simulink model "COM_BancMonitor"  (Simulink 8.6)
settings: Solver=FixedStepDiscrete  StartTime=0.0  StopTime=inf  FixedStep=ComMinSampleTime  RelTol=1e-3
values from neighbouring files (symbols this model uses):
  ComMinSampleTime = 1/400    (= 0.0025)    [init_BancMonitor.m]
  g = 9.81    [init_BancMonitor.m]
  LandingHeight = 0.08    [init_BancMonitor.m]
  Ts_AttitudeLoop = 1/200    (= 0.005)    [init_BancMonitor.m]
  Ts_PositionLoop = 1/100    (= 0.01)    [init_BancMonitor.m]
undefined symbols (not defined in the file or in its folder): a_PWM, b_PWM, BiasAcc, DiscIntNeverNeededParam, Gumstix, m, MaxThrottle, MinThrottle, MPU6050, PositionSecuMax, PositionSecuMin, Tacc, time_unfolding, Tmax, Tmin, TorquesSat, UAVstruct
undefined symbols (not defined in the file): AccMax, AccMaxScenario, AccMin, AccMinScenario, b_est0, dc_open, PositionMax, PositionMin, SpeedMax, SpeedMaxScenario, SpeedMin, SpeedMinScenario, Ts_detector, Ts_Wifi
libraries: simulink x34, custom_lib x27, simulink_extras x11
(part 2 of 3)

== system COM_BancMonitor/GUMSTIX/DETECTOR_PARAMETERS ==
  Max_no_detection : Constant  Value=5  OutDataTypeStr=Inherit: Inherit via back propagation  SampleTime=-1
  Mux6 : Mux  Inputs=[2 2 2 4 2 4 2 4]
  bin_square : Constant  Value=100  OutDataTypeStr=Inherit: Inherit via back propagation  SampleTime=-1
  blur_size : Constant  Value=3  OutDataTypeStr=Inherit: Inherit via back propagation  SampleTime=-1
  float32 to uint8 (BE) : custom_lib/CONVERTERS/float32 to uint8 (BE)
  float32 to uint8 (BE)1 : custom_lib/CONVERTERS/float32 to uint8 (BE)
  float32 to uint8 (BE)2 : custom_lib/CONVERTERS/float32 to uint8 (BE)
  k_approx : Constant  Value=0.02  OutDataTypeStr=Inherit: Inherit via back propagation  SampleTime=-1
  thresh_area : Constant  Value=1000  OutDataTypeStr=Inherit: Inherit via back propagation  SampleTime=-1
  thresh_cos : Constant  Value=0.1  OutDataTypeStr=Inherit: Inherit via back propagation  SampleTime=-1
  thresh_diff : Constant  Value=20*20  OutDataTypeStr=Inherit: Inherit via back propagation  SampleTime=-1
  thresh_ratio : Constant  Value=0.2  OutDataTypeStr=Inherit: Inherit via back propagation  SampleTime=-1
  uint16 to uint8 (BE){,1..4} (5 alike) : custom_lib/CONVERTERS/uint16 to uint8 (BE)
  Detector_param : Outport
  wires:
  Mux6/1 -> Detector_param/1
  thresh_ratio/1 -> float32 to uint8 (BE)2/1
  k_approx/1 -> float32 to uint8 (BE)/1
  thresh_area/1 -> uint16 to uint8 (BE)2/1
  thresh_cos/1 -> float32 to uint8 (BE)1/1
  thresh_diff/1 -> uint16 to uint8 (BE)3/1
  float32 to uint8 (BE)/1 -> Mux6/4
  float32 to uint8 (BE)1/1 -> Mux6/6
  float32 to uint8 (BE)2/1 -> Mux6/8
  blur_size/1 -> uint16 to uint8 (BE)1/1
  bin_square/1 -> uint16 to uint8 (BE)/1
  uint16 to uint8 (BE)2/1 -> Mux6/5
  uint16 to uint8 (BE)3/1 -> Mux6/7
  uint16 to uint8 (BE)1/1 -> Mux6/2
  uint16 to uint8 (BE)/1 -> Mux6/3
  Max_no_detection/1 -> uint16 to uint8 (BE)4/1
  uint16 to uint8 (BE)4/1 -> Mux6/1

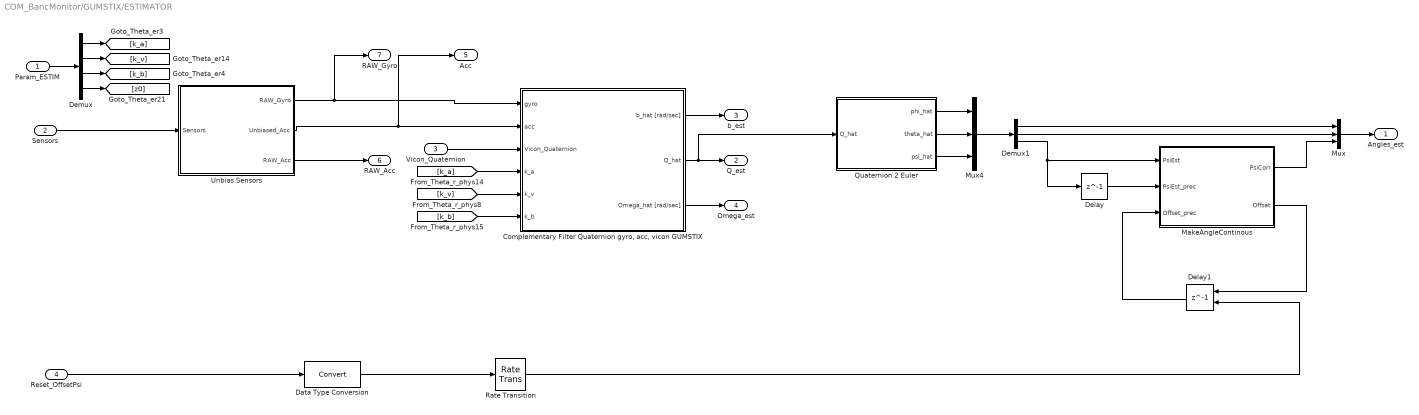
== system COM_BancMonitor/GUMSTIX/ESTIMATOR ==
  Param_ESTIM : Inport
  Sensors : Inport  Port=2
  Vicon_Quaternion : Inport  Port=3
  Reset_OffsetPsi : Inport  Port=4
  "Complementary Filter Quaternion gyro, acc, vicon GUMSTIX" : Subsystem  mask(COMPLEMENTARY FILTER){Ts_param=Ts_AttitudeLoop, b0_param=single(b_est0), Q0_param=single([1;0;0;0]), acc_ref_param=single([0;0;-g])}
      mask prompts: Ts_param "Sample Time [s]"; b0_param "Initial bias [deg/s]"; Q0_param "Initial Quaternion"; acc_ref_param "Accelerometer Reference"
      mask help:
      | This block assure a complementary filtering of IMU's data and vicon's data.
      |
      | ka: the gain to adjust accelerometer's sensibility
      |     A digonal matrix [3x3]:
      | kv: the gain to adjust vicon's sensibility
      |     A digonal matrix [3x3]
      | kb: the gain to adjust the bias sensibility
      |     A digonal matrix [3x3]
      |
      | Remark: For each diagonal matrix gain:
      |     - kx(1,1) = roll sensibilty
      |     - kx(2,2) = pitch sensibilty
      |     - kx(3,3) = yaw sensibilty
  Data Type Conversion : DataTypeConversion
  Delay : Delay  DelayLength=1
  Delay1 : Delay  DelayLength=1  ExternalReset=Level hold
      settings: InputPortMap=u0,r5
  Demux : Demux  Outputs=[3; 3; 3; 1]
  Demux1 : Demux  Outputs=3
  MakeAngleContinous : MATLAB Function  TreatAsAtomicUnit=on
  Mux : Mux  Inputs=3
  Mux4 : Mux  Inputs=3
  Quaternion 2 Euler : MATLAB Function  TreatAsAtomicUnit=on
  Rate Transition : RateTransition
  Unbias Sensors : Subsystem
  Angles_est : Outport
  Q_est : Outport  Port=2
  b_est : Outport  Port=3
  Omega_est : Outport  Port=4
  Acc : Outport  Port=5
  RAW_Acc : Outport  Port=6
  RAW_Gyro : Outport  Port=7
  wires:
  Sensors/1 -> Unbias Sensors/1(Sensors)
  Unbias Sensors/2(Unbiased_Acc) -> Acc/1, "Complementary Filter Quaternion gyro, acc, vicon GUMSTIX"/2(acc)
  Unbias Sensors/1(RAW_Gyro) -> "Complementary Filter Quaternion gyro, acc, vicon GUMSTIX"/1(gyro), RAW_Gyro/1
  "Complementary Filter Quaternion gyro, acc, vicon GUMSTIX"/1(b_hat [rad/sec]) -> b_est/1
  [k_a] -> "Complementary Filter Quaternion gyro, acc, vicon GUMSTIX"/4(k_a)
  "Complementary Filter Quaternion gyro, acc, vicon GUMSTIX"/2(Q_hat) -> Q_est/1, Quaternion 2 Euler/1(Q_hat)
  [k_v] -> "Complementary Filter Quaternion gyro, acc, vicon GUMSTIX"/5(k_v)
  [k_b] -> "Complementary Filter Quaternion gyro, acc, vicon GUMSTIX"/6(k_b)
  Param_ESTIM/1 -> Demux/1
  Demux/1 -> [k_a]
  Demux/2 -> [k_v]
  Demux/3 -> [k_b]
  Demux/4 -> [z0]
  Vicon_Quaternion/1 -> "Complementary Filter Quaternion gyro, acc, vicon GUMSTIX"/3(Vicon_Quaternion)
  Delay/1 -> MakeAngleContinous/2(PsiEst_prec)
  Delay1/1 -> MakeAngleContinous/3(Offset_prec)
  MakeAngleContinous/2(Offset) -> Delay1/1
  Mux/1 -> Angles_est/1
  Demux1/3 -> Delay/1, MakeAngleContinous/1(PsiEst)
  Demux1/2 -> Mux/2
  Demux1/1 -> Mux/1
  MakeAngleContinous/1(PsiCorr) -> Mux/3
  Reset_OffsetPsi/1 -> Data Type Conversion/1
  Rate Transition/1 -> Delay1/2
  Data Type Conversion/1 -> Rate Transition/1
  Unbias Sensors/3(RAW_Acc) -> RAW_Acc/1
  Quaternion 2 Euler/1(phi_hat) -> Mux4/1
  Quaternion 2 Euler/2(theta_hat) -> Mux4/2
  Quaternion 2 Euler/3(psi_hat) -> Mux4/3
  Mux4/1 -> Demux1/1
  "Complementary Filter Quaternion gyro, acc, vicon GUMSTIX"/3(Omega_hat [rad/sec]) -> Omega_est/1

== system COM_BancMonitor/GUMSTIX/ESTIMATOR_PARAMETERS ==
  Mux1 : Mux  Inputs=2
  Mux6 : Mux  Inputs=3
  Time Constant Gyro Filter : Constant  Value=0.3897 %exp(-2*pi*30*ComMinSampleTime)  OutDataTypeStr=Inherit: Inherit via back propagation  SampleTime=-1
  k_a : Constant  Value=[.4 .4 0]  OutDataTypeStr=Inherit: Inherit via back propagation  SampleTime=-1
  k_b : Constant  Value=[.08 .08 .08]  OutDataTypeStr=Inherit: Inherit via back propagation  SampleTime=-1
  k_v : Constant  Value=[0 0 2]  OutDataTypeStr=Inherit: Inherit via back propagation  SampleTime=-1
  Est_Param : Outport
  wires:
  k_a/1 -> Mux6/1
  k_b/1 -> Mux6/3
  k_v/1 -> Mux6/2
  Mux6/1 -> Mux1/1
  Time Constant Gyro Filter/1 -> Mux1/2
  Mux1/1 -> Est_Param/1

== system COM_BancMonitor/GUMSTIX/Manual_Controller ==
  RX_Data : Inport
  Angles_est : Inport  Port=2
  Gyo Acc2 : Mux  Inputs=[1 1 1]
  In_from_UDP_Demux1 : Demux  Outputs=3
  In_from_UDP_Demux3 : Demux  Outputs=[1 1 1 1]
  Product : Product  Inputs=*/  RndMeth=Zero
  Product1 : Product  Inputs=**  RndMeth=Zero
  RX Angles Ref  Generator : Subsystem
  Saturation1 : Saturate  UpperLimit=Tmax*9.81*4  LowerLimit=Tmin*9.81*4
  Terminator : Terminator
  Trigonometric Function : Trigonometry  Operator=cos
  Trigonometric Function1 : Trigonometry  Operator=cos
  Angles_ref : Outport
  Thrust_ref : Outport  Port=2
  wires:
  RX Angles Ref  Generator/1(Roll_ref) -> Gyo Acc2/1
  RX Angles Ref  Generator/2(Pitch_ref) -> Gyo Acc2/2
  RX Angles Ref  Generator/3(Yaw_ref) -> Gyo Acc2/3
  Angles_est/1 -> In_from_UDP_Demux1/1
  Product1/1 -> Product/2
  In_from_UDP_Demux1/1 -> Trigonometric Function/1
  In_from_UDP_Demux1/2 -> Trigonometric Function1/1
  In_from_UDP_Demux1/3 -> Terminator/1
  Trigonometric Function1/1 -> Product1/2
  Trigonometric Function/1 -> Product1/1
  RX Angles Ref  Generator/4(Throttle_ref) -> Product/1
  Product/1 -> Saturation1/1
  Saturation1/1 -> Thrust_ref/1
  In_from_UDP_Demux3/1 -> RX Angles Ref  Generator/1(Roll_RX)
  In_from_UDP_Demux3/2 -> RX Angles Ref  Generator/2(Pitch_RX)
  In_from_UDP_Demux3/3 -> RX Angles Ref  Generator/3(Yaw_RX)
  In_from_UDP_Demux3/4 -> RX Angles Ref  Generator/4(Throttle_RX)
  RX_Data/1 -> In_from_UDP_Demux3/1
  Gyo Acc2/1 -> Angles_ref/1

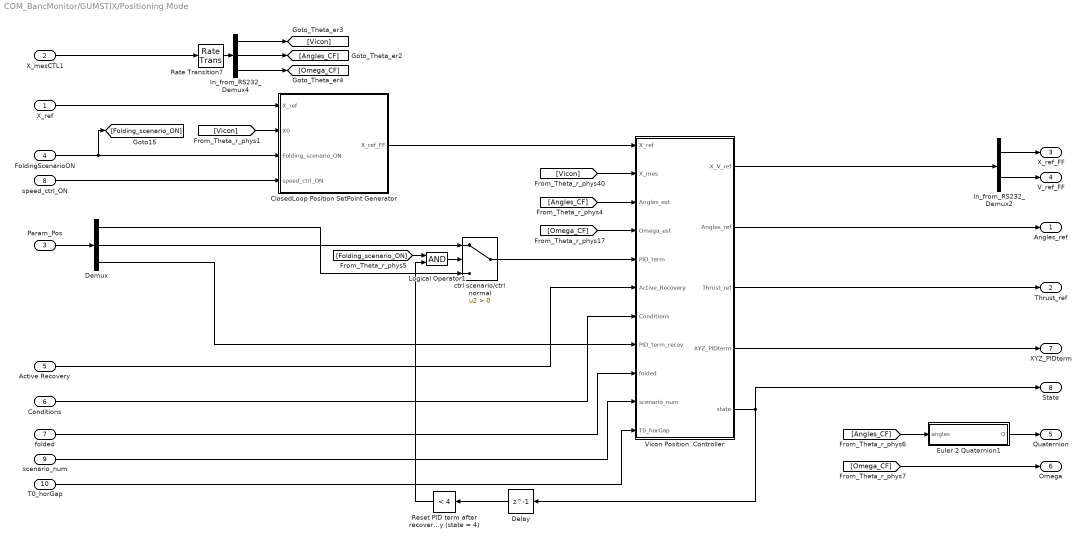
== system COM_BancMonitor/GUMSTIX/Positioning Mode ==
  X_ref : Inport
  X_mesCTL1 : Inport  Port=2
  Param_Pos : Inport  Port=3
  FoldingScenarioON : Inport  Port=4
  Active Recovery : Inport  Port=5
  Conditions : Inport  Port=6
  folded : Inport  Port=7
  speed_ctrl_ON : Inport  Port=8
  scenario_num : Inport  Port=9
  T0_horGap : Inport  Port=10
  ClosedLoop Position SetPoint Generator : Subsystem
  Delay : Delay  DelayLength=1  InitialCondition=0
  Demux : Demux  Outputs=[12 12 12]
  Euler 2 Quaternion1 : MATLAB Function  TreatAsAtomicUnit=on
  In_from_RS232_Demux2 : Demux  Outputs=[3 3]
  In_from_RS232_Demux4 : Demux  Outputs=[6 3 3]
  Logical Operator1 : Logic  AllPortsSameDT=off  OutDataTypeStr=boolean
  Rate Transition7 : RateTransition  OutPortSampleTime=Ts_PositionLoop
  Reset PID term after recovery (state = 4) : simulink/Logic and Bit Operations/Compare To Constant  relop=<  const=4  OutDataTypeStr=boolean
  Vicon Position  Controller : Subsystem
  ctrl scenario/ctrl normal : Switch  Criteria=u2 > Threshold
  Angles_ref : Outport
  Thrust_ref : Outport  Port=2
  X_ref_FF : Outport  Port=3
  V_ref_FF : Outport  Port=4
  Quaternion : Outport  Port=5
  Omega : Outport  Port=6
  XYZ_PIDterm : Outport  Port=7
  State : Outport  Port=8
  wires:
  [Vicon] -> Vicon Position  Controller/2(X_mes)
  [Vicon] -> ClosedLoop Position SetPoint Generator/2(X0)
  ClosedLoop Position SetPoint Generator/1(X_ref_FF) -> Vicon Position  Controller/1(X_ref)
  In_from_RS232_Demux2/1 -> X_ref_FF/1
  In_from_RS232_Demux2/2 -> V_ref_FF/1
  Vicon Position  Controller/1(X_V_ref) -> In_from_RS232_Demux2/1
  In_from_RS232_Demux4/1 -> [Vicon]
  In_from_RS232_Demux4/2 -> [Angles_CF]
  [Angles_CF] -> Vicon Position  Controller/3(Angles_est)
  Euler 2 Quaternion1/1(Q) -> Quaternion/1
  [Omega_CF] -> Omega/1
  In_from_RS232_Demux4/3 -> [Omega_CF]
  X_mesCTL1/1 -> Rate Transition7/1
  Rate Transition7/1 -> In_from_RS232_Demux4/1
  Vicon Position  Controller/4(XYZ_PIDterm) -> XYZ_PIDterm/1
  FoldingScenarioON/1 -> ClosedLoop Position SetPoint Generator/3(Folding_scenario_ON), [Folding_scenario_ON]
  X_ref/1 -> ClosedLoop Position SetPoint Generator/1(X_ref)
  Vicon Position  Controller/3(Thrust_ref) -> Thrust_ref/1
  [Omega_CF] -> Vicon Position  Controller/4(Omega_est)
  Vicon Position  Controller/2(Angles_ref) -> Angles_ref/1
  Vicon Position  Controller/5(state) -> State/1, Delay/1
  Param_Pos/1 -> Demux/1
  Demux/3 -> Vicon Position  Controller/8(PID_term_recov)
  Active Recovery/1 -> Vicon Position  Controller/6(Active_Recovery)
  Demux/2 -> ctrl scenario/ctrl normal/1
  ctrl scenario/ctrl normal/1 -> Vicon Position  Controller/5(PID_term)
  Demux/1 -> ctrl scenario/ctrl normal/3
  Conditions/1 -> Vicon Position  Controller/7(Conditions)
  [Folding_scenario_ON] -> Logical Operator1/1
  Logical Operator1/1 -> ctrl scenario/ctrl normal/2
  Reset PID term after recovery (state = 4)/1 -> Logical Operator1/2
  Delay/1 -> Reset PID term after recovery (state = 4)/1
  folded/1 -> Vicon Position  Controller/9(folded)
  speed_ctrl_ON/1 -> ClosedLoop Position SetPoint Generator/4(speed_ctrl_ON)
  scenario_num/1 -> Vicon Position  Controller/10(scenario_num)
  [Angles_CF] -> Euler 2 Quaternion1/1(angles)
  T0_horGap/1 -> Vicon Position  Controller/11(T0_horGap)

== system COM_BancMonitor/GUMSTIX/Torques  Disturbances ==
  Torques : Inport
  Dist_Torques : Inport  Port=2
  " " : Constant  Value=[0 0 0]  OutDataTypeStr=Inherit: Inherit via back propagation
  Add : Sum
  Add1 : Sum
  Add2 : Sum
  Compare To Constant : simulink/Logic and Bit Operations/Compare To Constant  relop===  const=1  OutDataTypeStr=boolean
  Compare To Constant1 : simulink/Logic and Bit Operations/Compare To Constant  relop===  const=3  OutDataTypeStr=boolean
  Demux2 : Demux  Outputs=3
  Demux3 : Demux  Outputs=3
  Multiport Switch : MultiPortSwitch  DataPortForDefault=Additional data port
  Mux : Mux  Inputs=3
  Mux1 : Mux  Inputs=3
  Selector : Selector  InputPortWidth=5  IndexOptions=Index vector (dialog)  Indices=[1 2 3]  OutputSizes=1
  Selector2 : Selector  InputPortWidth=5  IndexOptions=Index vector (dialog)  Indices=4  OutputSizes=1
  Selector3 : Selector  InputPortWidth=5  IndexOptions=Index vector (dialog)  Indices=5  OutputSizes=1
  Triggered Subsystem : Subsystem  TreatAsAtomicUnit=on
  Triggered Subsystem1 : Subsystem  TreatAsAtomicUnit=on
  Torques_Out : Outport
  dist_torques_OUT : Outport  Port=2
  wires:
  Dist_Torques/1 -> Selector2/1, Selector3/1, Selector/1
  Selector/1 -> Triggered Subsystem1/1(TorquesDist Mag), Multiport Switch/3, Triggered Subsystem/1(TorquesDist Mag)
  Selector3/1 -> Mux1/3, Multiport Switch/1, Compare To Constant1/1, Compare To Constant/1
  Demux2/1 -> Add/1
  Demux2/2 -> Add1/1
  Demux2/3 -> Add2/1
  Add/1 -> Mux/1
  Add1/1 -> Mux/2
  Add2/1 -> Mux/3
  Demux3/2 -> Add1/2
  Demux3/1 -> Add/2
  Demux3/3 -> Add2/2
  Selector2/1 -> Mux1/2, Triggered Subsystem1/2(Dt), Triggered Subsystem/2(Dt)
  Torques/1 -> Demux2/1
  Mux/1 -> Torques_Out/1
  Compare To Constant/1 -> Triggered Subsystem/Enable
  Triggered Subsystem/1(DisturbTorques) -> Multiport Switch/2
  Multiport Switch/1 -> Demux3/1, Mux1/1
  " "/1 -> Multiport Switch/5
  Compare To Constant1/1 -> Triggered Subsystem1/Enable
  Triggered Subsystem1/1(DisturbTorques) -> Multiport Switch/4
  Mux1/1 -> dist_torques_OUT/1

== system COM_BancMonitor/GUMSTIX/Torques saturation ==
  Torques : Inport
  gamma [deg] : Inport  Port=2
  Constant : Constant  Value=TorquesSat
  Convert : DataTypeConversion  RndMeth=Nearest
  Demux : Demux  Outputs=3
  Demux1 : Demux  Outputs=3
  Gain : Gain  Gain=-1
  Gain1 : Gain  Gain=-1
  Gain2 : Gain  Gain=-1
  MATLAB Function : MATLAB Function  TreatAsAtomicUnit=on
  Mux4 : Mux  Inputs=3
  Saturation Dynamic : simulink/Discontinuities/Saturation Dynamic  OutMin=[]  OutMax=[]  OutDataTypeStr=Inherit: Same as second input  OutDataType=fixdt(1, 16)  OutScaling=2^-10  DoSatur=off
  Saturation Dynamic1 : simulink/Discontinuities/Saturation Dynamic  OutMin=[]  OutMax=[]  OutDataTypeStr=Inherit: Same as second input  OutDataType=fixdt(1, 16)  OutScaling=2^-10  DoSatur=off
  Saturation Dynamic2 : simulink/Discontinuities/Saturation Dynamic  OutMin=[]  OutMax=[]  OutDataTypeStr=Inherit: Same as second input  OutDataType=fixdt(1, 16)  OutScaling=2^-10  DoSatur=off
  Torques_Sat : Outport
  Sats : Outport  Port=2
  wires:
  Mux4/1 -> Convert/1
  gamma [deg]/1 -> MATLAB Function/2(gamma)
  Constant/1 -> MATLAB Function/1(TorquesSat)
  Demux/1 -> Saturation Dynamic/2
  Demux/2 -> Saturation Dynamic1/2
  Demux/3 -> Saturation Dynamic2/2
  Saturation Dynamic/1 -> Mux4/1
  Saturation Dynamic1/1 -> Mux4/2
  Saturation Dynamic2/1 -> Mux4/3
  Torques/1 -> Demux/1
  Demux1/1 -> Gain/1, Saturation Dynamic/1
  Demux1/2 -> Gain1/1, Saturation Dynamic1/1
  Demux1/3 -> Gain2/1, Saturation Dynamic2/1
  Gain/1 -> Saturation Dynamic/3
  Gain1/1 -> Saturation Dynamic1/3
  Gain2/1 -> Saturation Dynamic2/3
  MATLAB Function/1(TSat) -> Sats/1, Demux1/1
  Convert/1 -> Torques_Sat/1

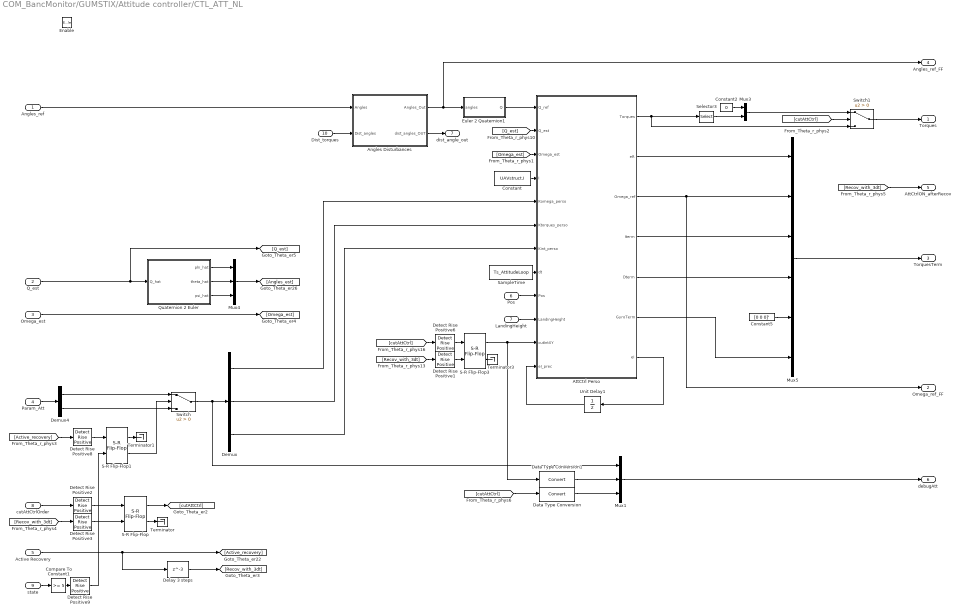
== system COM_BancMonitor/GUMSTIX/Attitude controller/CTL_ATT_NL ==
  Angles_ref : Inport
  Q_est : Inport  Port=2
  Omega_est : Inport  Port=3
  Param_Att : Inport  Port=4
  Active Recovery : Inport  Port=5
  Pos : Inport  Port=6
  LandingHeight : Inport  Port=7
  cutAttCtrlOrder : Inport  Port=8
  state : Inport  Port=9
  Dist_torques : Inport  Port=10
  Enable : EnablePort  StatesWhenEnabling=reset
  Angles Disturbances : Subsystem
  AttCtrl Perso : MATLAB Function  TreatAsAtomicUnit=on
  Compare To Constant1 : simulink/Logic and Bit Operations/Compare To Constant  relop=>=  const=5  OutDataTypeStr=boolean
  Constant : Constant  Value=UAVstruct.I  OutDataTypeStr=Inherit: Inherit via back propagation
  Constant2 : Constant  Value=0  OutDataTypeStr=Inherit: Inherit via back propagation
  Constant5 : Constant  Value=[0 0 0]'  OutDataTypeStr=Inherit: Inherit via back propagation
  Data Type Conversion : DataTypeConversion
  Data Type Conversion1 : DataTypeConversion
  Delay 3 steps : Delay  DelayLength=3  InitialCondition=0
  Demux : Demux  Outputs=[3 3 3]
  Demux4 : Demux  Outputs=2
  Detect Rise Positive{1..3,6,8..9} (6 alike) : simulink/Logic and Bit Operations/Detect Rise Positive  vinit=1  InputProcessing=Inherited  OutDataTypeStr=boolean
  Euler 2 Quaternion1 : MATLAB Function  TreatAsAtomicUnit=on
  Mux1 : Mux  Inputs=[9 1 1]
  Mux3 : Mux  Inputs=[1 2]
  Mux4 : Mux  Inputs=3
  Mux5 : Mux  Inputs=[3 3 3 3 3 3]
  Quaternion 2 Euler : MATLAB Function  TreatAsAtomicUnit=on
  S-R Flip-Flop : simulink_extras/Flip Flops/S-R Flip-Flop  initial_condition=0
  S-R Flip-Flop1 : simulink_extras/Flip Flops/S-R Flip-Flop  initial_condition=0
  S-R Flip-Flop3 : simulink_extras/Flip Flops/S-R Flip-Flop  initial_condition=0
  SampleTime : Constant  Value=Ts_AttitudeLoop  OutDataTypeStr=single  SampleTime=-1
  Selector3 : Selector  InputPortWidth=3  IndexOptions=Index vector (dialog)  Indices=[2 3]  OutputSizes=1
  Switch : Switch  Criteria=u2 > Threshold
  Switch1 : Switch  Criteria=u2 > Threshold
  Terminator : Terminator
  Terminator1 : Terminator
  Terminator3 : Terminator
  Unit Delay1 : UnitDelay  InitialCondition=single([0 0 0])  SampleTime=-1
  Torques : Outport  InitialOutput=[0; 0; 0]
  Omega_ref_FF : Outport  Port=2  InitialOutput=[0; 0; 0]
  TorquesTerm : Outport  Port=3  InitialOutput=zeros(18, 1)
  Angles_ref_FF : Outport  Port=4  InitialOutput=[0; 0; 0]
  AttCtrlON_afterRecov : Outport  Port=5  InitialOutput=0
  debugAtt : Outport  Port=6  InitialOutput=zeros(11,0)
  dist_angle_out : Outport  Port=7  InitialOutput=[0; 0; 0; 0; 0]
  wires:
  Constant2/1 -> Mux3/1
  Mux3/1 -> Switch1/1
  [cutAttCtrl] -> Switch1/2
  Active Recovery/1 -> Delay 3 steps/1, [Active_recovery]
  Delay 3 steps/1 -> [Recov_with_3dt]
  [Recov_with_3dt] -> Detect Rise Positive3/1
  [Recov_with_3dt] -> AttCtrlON_afterRecov/1
  Q_est/1 -> [Q_est], Quaternion 2 Euler/1(Q_hat)
  Omega_est/1 -> [Omega_est]
  Quaternion 2 Euler/1(phi_hat) -> Mux4/1
  Quaternion 2 Euler/2(theta_hat) -> Mux4/2
  Quaternion 2 Euler/3(psi_hat) -> Mux4/3
  Mux4/1 -> [Angles_est]
  cutAttCtrlOrder/1 -> Detect Rise Positive2/1
  S-R Flip-Flop/1 -> [cutAttCtrl]
  S-R Flip-Flop/2 -> Terminator/1
  Detect Rise Positive2/1 -> S-R Flip-Flop/1
  Detect Rise Positive3/1 -> S-R Flip-Flop/2
  Demux/1 -> AttCtrl Perso/5(Komega_perso)
  Demux/2 -> AttCtrl Perso/6(Ktorques_perso)
  Euler 2 Quaternion1/1(Q) -> AttCtrl Perso/1(Q_ref)
  AttCtrl Perso/1(Torques) -> Switch1/3, Selector3/1
  AttCtrl Perso/2(eR) -> Mux5/1
  AttCtrl Perso/6(GyroTerm) -> Mux5/6
  Mux5/1 -> TorquesTerm/1
  AttCtrl Perso/3(Omega_ref) -> Omega_ref_FF/1, Mux5/2
  AttCtrl Perso/7(eI) -> Unit Delay1/1
  Unit Delay1/1 -> AttCtrl Perso/12(eI_prec)
  AttCtrl Perso/4(Iterm) -> Mux5/3
  Demux/3 -> AttCtrl Perso/7(Kint_perso)
  Switch1/1 -> Torques/1
  state/1 -> Compare To Constant1/1
  AttCtrl Perso/5(Dterm) -> Mux5/4
  S-R Flip-Flop3/1 -> Data Type Conversion1/1, AttCtrl Perso/11(cutIntXY)
  S-R Flip-Flop3/2 -> Terminator3/1
  [cutAttCtrl] -> Detect Rise Positive6/1
  Detect Rise Positive6/1 -> S-R Flip-Flop3/1
  Detect Rise Positive1/1 -> S-R Flip-Flop3/2
  Constant5/1 -> Mux5/5
  [Recov_with_3dt] -> Detect Rise Positive1/1
  Constant/1 -> AttCtrl Perso/4(I)
  SampleTime/1 -> AttCtrl Perso/8(dt)
  Pos/1 -> AttCtrl Perso/9(Pos)
  LandingHeight/1 -> AttCtrl Perso/10(LandingHeight)
  [Omega_est] -> AttCtrl Perso/3(Omega_est)
  Param_Att/1 -> Demux4/1
  Demux4/1 -> Switch/1
  Demux4/2 -> Switch/3
  Switch/1 -> Mux1/1, Demux/1
  [Active_recovery] -> Detect Rise Positive8/1
  Detect Rise Positive8/1 -> S-R Flip-Flop1/1
  S-R Flip-Flop1/1 -> Terminator1/1
  S-R Flip-Flop1/2 -> Switch/2
  Compare To Constant1/1 -> Detect Rise Positive9/1
  Detect Rise Positive9/1 -> S-R Flip-Flop1/2
  [cutAttCtrl] -> Data Type Conversion/1
  Mux1/1 -> debugAtt/1
  Data Type Conversion/1 -> Mux1/3
  Data Type Conversion1/1 -> Mux1/2
  Angles Disturbances/1(Angles_Out) -> Angles_ref_FF/1, Euler 2 Quaternion1/1(angles)
  Angles Disturbances/2(dist_angles_OUT) -> dist_angle_out/1
  Dist_torques/1 -> Angles Disturbances/2(Dist_angles)
  [Q_est] -> AttCtrl Perso/2(Q_est)
  Angles_ref/1 -> Angles Disturbances/1(Angles)
  Selector3/1 -> Mux3/2

== system COM_BancMonitor/GUMSTIX/Control Mix/Control_mix ==
  Thrust : Inport
  Torques : Inport  Port=2
  gamma [deg] : Inport  Port=3
  Constant : Constant  Value=UAVstruct.iGamma  OutDataTypeStr=Inherit: Inherit via back propagation
  Demux : Demux
  Mixage : MATLAB Function  TreatAsAtomicUnit=on
  Mux1 : Mux  Inputs=2
  Rate Transition : RateTransition
  Saturation1 : Saturate  UpperLimit=inf  LowerLimit=0
  Sqrt1 : Sqrt  SaturateOnIntegerOverflow=on
  omega_r1_ref : Outport
  omega_r2_ref : Outport  Port=2
  omega_r3_ref : Outport  Port=3
  omega_r4_ref : Outport  Port=4
  wires:
  Demux/1 -> omega_r1_ref/1
  Demux/2 -> omega_r2_ref/1
  Demux/3 -> omega_r3_ref/1
  Demux/4 -> omega_r4_ref/1
  Sqrt1/1 -> Rate Transition/1
  Rate Transition/1 -> Demux/1
  Thrust/1 -> Mux1/1
  Torques/1 -> Mux1/2
  Mixage/1(omega2) -> Saturation1/1
  Saturation1/1 -> Sqrt1/1
  gamma [deg]/1 -> Mixage/3(gamma)
  Mux1/1 -> Mixage/2(ThrustTorques)
  Constant/1 -> Mixage/1(iGamma)

== system COM_BancMonitor/GUMSTIX/Control Mix/Omega_ref 2 PWM_ref ==
  Omega_ref : Inport
  Bias : Bias  Bias=b_PWM
  Gain : Gain  Gain=a_PWM
  PWM_ref : Outport
  wires:
  Gain/1 -> Bias/1
  Bias/1 -> PWM_ref/1
  Omega_ref/1 -> Gain/1

== system COM_BancMonitor/GUMSTIX/ESTIMATOR/Complementary Filter Quaternion gyro, acc, vicon GUMSTIX ==
  gyro : Inport
  acc : Inport  Port=2
  Vicon_Quaternion : Inport  Port=3
  k_a : Inport  Port=4
  k_v : Inport  Port=5
  k_b : Inport  Port=6
  Attitude_Est : MATLAB Function  TreatAsAtomicUnit=on
  Bias : Delay  DelayLength=1  InitialCondition=b0_param  SampleTime=Ts_param
  Constant1 : Constant  Value=Ts_param  OutDataTypeStr=Inherit: Inherit via back propagation
  Constant7 : Constant  Value=acc_ref_param  VectorParams1D=off  OutDataTypeStr=Inherit: Inherit via back propagation
  Quaternion : Delay  DelayLength=1  InitialCondition=Q0_param  SampleTime=Ts_param
  b_hat [rad/sec] : Outport
  Q_hat : Outport  Port=2
  Omega_hat [rad/sec] : Outport  Port=3
  wires:
  Attitude_Est/1(Q_hat) -> Q_hat/1, Quaternion/1
  Attitude_Est/2(b_hat) -> Bias/1, b_hat [rad/sec]/1
  Constant1/1 -> Attitude_Est/6(dt)
  Bias/1 -> Attitude_Est/2(b_hat_prec)
  Quaternion/1 -> Attitude_Est/1(Q_hat_prec)
  Attitude_Est/3(Omega_hat) -> Omega_hat [rad/sec]/1
  acc/1 -> Attitude_Est/4(acc_imu)
  gyro/1 -> Attitude_Est/3(gyro_imu)
  Constant7/1 -> Attitude_Est/10(acc_ref)
  Vicon_Quaternion/1 -> Attitude_Est/5(Q_Vicon)
  k_a/1 -> Attitude_Est/7(k_a)
  k_v/1 -> Attitude_Est/8(k_v)
  k_b/1 -> Attitude_Est/9(k_b)

== system COM_BancMonitor/GUMSTIX/ESTIMATOR/Unbias Sensors ==
  Sensors : Inport
  Bias : Bias  Bias=-BiasAcc
  Constant : Constant  Value=single(Tacc)
  Demux2 : Demux  Outputs=[3 3]
  Product : Product  Multiplication=Matrix(*)  RndMeth=Zero
  int16_2_g : Gain  Gain=MPU6050.acc.int16_2_g  OutDataTypeStr=Inherit: Same as input
  int16_2_rad : Gain  Gain=MPU6050.gyr.int16_2_rad  OutDataTypeStr=Inherit: Same as input
  RAW_Gyro : Outport
  Unbiased_Acc : Outport  Port=2
  RAW_Acc : Outport  Port=3
  wires:
  Sensors/1 -> Demux2/1
  int16_2_g/1 -> RAW_Acc/1, Bias/1
  Demux2/1 -> int16_2_rad/1
  int16_2_rad/1 -> RAW_Gyro/1
  Demux2/2 -> int16_2_g/1
  Bias/1 -> Product/2
  Constant/1 -> Product/1
  Product/1 -> Unbiased_Acc/1

== system COM_BancMonitor/GUMSTIX/Manual_Controller/RX Angles Ref  Generator ==
  Roll_RX : Inport
  Pitch_RX : Inport  Port=2
  Yaw_RX : Inport  Port=3
  Throttle_RX : Inport  Port=4
  Rescale Pitch : Subsystem  mask{MinInput=1000, MaxInput=2000, DeadZone=10, MinOutput=-20*pi/180, MaxOutput=20*pi/180, G_Scale=0, BiasScale=0}
      mask prompts: MinInput "Minimum Input"; MaxInput "Maximum Input"; DeadZone "Dead Zone"; MinOutput "Minimum Output"; MaxOutput "Maximum Output"; BiasScale "Bias_Scale"
      mask init:
      | Gscale = (MaxOutput-MinOutput)/(MaxInput-MinInput-2*DeadZone);
      | Bias_Scale = MinInput+(MaxInput-MinInput)/2;
  Rescale Roll : Subsystem  mask{MinInput=1000, MaxInput=2000, DeadZone=10, MinOutput=-20*pi/180, MaxOutput=20*pi/180, G_Scale=0, BiasScale=0}
      mask prompts: MinInput "Minimum Input"; MaxInput "Maximum Input"; DeadZone "Dead Zone"; MinOutput "Minimum Output"; MaxOutput "Maximum Output"; BiasScale "Bias_Scale"
      mask init:
      | Gscale = (MaxOutput-MinOutput)/(MaxInput-MinInput-2*DeadZone);
      | Bias_Scale = MinInput+(MaxInput-MinInput)/2;
  Rescale Yaw : Subsystem  mask{MinInput=1000, MaxInput=2000, DeadZone=10, MinOutput=-30*pi/180, MaxOutput=30*pi/180, G_Scale=0, BiasScale=0}
      mask prompts: MinInput "Minimum Input"; MaxInput "Maximum Input"; DeadZone "Dead Zone"; MinOutput "Minimum Output"; MaxOutput "Maximum Output"; BiasScale "Bias_Scale"
      mask init:
      | Gscale = (MaxOutput-MinOutput)/(MaxInput-MinInput-2*DeadZone);
      | Bias_Scale = MinInput+(MaxInput-MinInput)/2;
  Rescale2 Throttle : Subsystem  mask{MinInput=1000, MaxInput=2000, MinOutput=0*m*g, MaxOutput=1.3*m*g, G_Scale=0}
      mask prompts: MinInput "Minimum Input"; MaxInput "Maximum Input"; MinOutput "Minimum Output"; MaxOutput "Maximum Output"
      mask init:
      | Gscale = (MaxOutput-MinOutput)/(MaxInput-MinInput);
  Roll_ref : Outport
  Pitch_ref : Outport  Port=2
  Yaw_ref : Outport  Port=3
  Throttle_ref : Outport  Port=4
  wires:
  Roll_RX/1 -> Rescale Roll/1(In)
  Pitch_RX/1 -> Rescale Pitch/1(In)
  Yaw_RX/1 -> Rescale Yaw/1(In)
  Rescale Roll/1(Out) -> Roll_ref/1
  Rescale Pitch/1(Out) -> Pitch_ref/1
  Rescale Yaw/1(Out) -> Yaw_ref/1
  Throttle_RX/1 -> Rescale2 Throttle/1(In)
  Rescale2 Throttle/1(Out) -> Throttle_ref/1

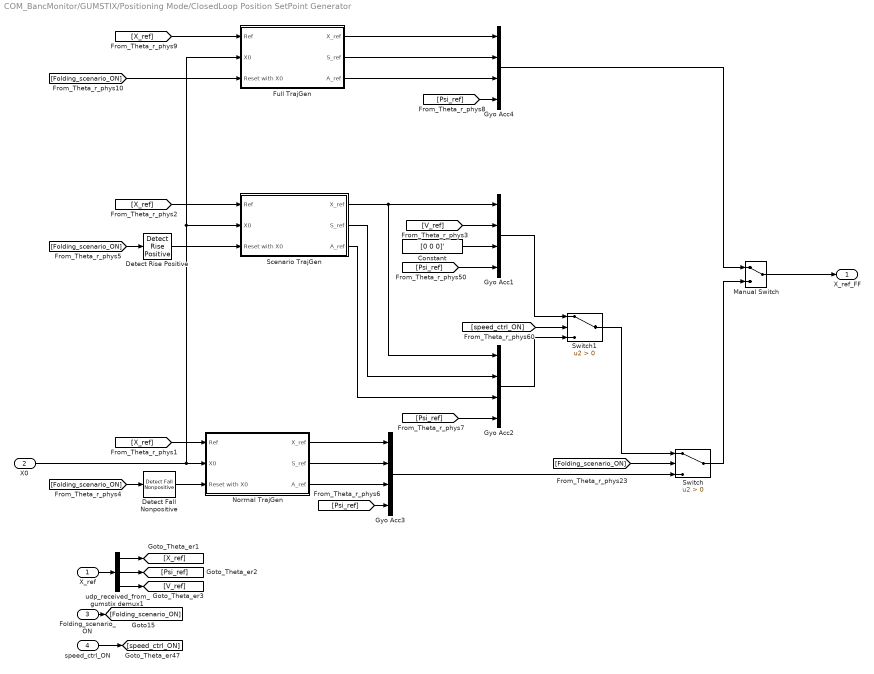
== system COM_BancMonitor/GUMSTIX/Positioning Mode/ClosedLoop Position SetPoint Generator ==
  X_ref : Inport
  X0 : Inport  Port=2
  Folding_scenario_ON : Inport  Port=3
  speed_ctrl_ON : Inport  Port=4
  Constant : Constant  Value=[0 0 0]'  OutDataTypeStr=Inherit: Inherit via back propagation
  Detect Fall Nonpositive : simulink/Logic and Bit Operations/Detect Fall Nonpositive  vinit=1  InputProcessing=Inherited  OutDataTypeStr=boolean
  Detect Rise Positive : simulink/Logic and Bit Operations/Detect Rise Positive  vinit=1  InputProcessing=Inherited  OutDataTypeStr=boolean
  Full TrajGen : Subsystem  mask{Tau=[3/6 3/6 5/6]', Ts_Filter=Ts_PositionLoop, Xmax=PositionMax, Xmin=PositionMin, Smax=SpeedMax, Smin=SpeedMin, Amax=AccMax, Amin=AccMin}
      mask prompts: Ts_Filter "Ts"; Xmax "Pos max"; Xmin "Pos min"; Smax "Speed max"; Smin "Speed min"; Amax "Acc max"; Amin "Acc min"
  Gyo Acc{1..4} (4 alike) : Mux
  Manual Switch : ManualSwitch
  Normal TrajGen : Subsystem  mask{Tau=[3/6 3/6 5/6]', Ts_Filter=Ts_PositionLoop, Xmax=PositionMax, Xmin=PositionMin, Smax=SpeedMax, Smin=SpeedMin, Amax=AccMax, Amin=AccMin}
      mask prompts: Ts_Filter "Ts"; Xmax "Pos max"; Xmin "Pos min"; Smax "Speed max"; Smin "Speed min"; Amax "Acc max"; Amin "Acc min"
  Scenario TrajGen : Subsystem  mask{Tau=[3/6 3/6 5/6]', Ts_Filter=Ts_PositionLoop, Xmax=PositionMax, Xmin=PositionMin, Smax=SpeedMaxScenario, Smin=SpeedMinScenario, Amax=AccMaxScenario, Amin=AccMinScenario}
      mask prompts: Ts_Filter "Ts"; Xmax "Pos max"; Xmin "Pos min"; Smax "Speed max"; Smin "Speed min"; Amax "Acc max"; Amin "Acc min"
  Switch : Switch  Criteria=u2 > Threshold
  Switch1 : Switch  Criteria=u2 > Threshold
  udp_received_from_gumstix demux1 : Demux  Outputs=[3 1 3]
  X_ref_FF : Outport
  wires:
  [X_ref] -> Normal TrajGen/1(Ref)
  udp_received_from_gumstix demux1/1 -> [X_ref]
  udp_received_from_gumstix demux1/2 -> [Psi_ref]
  X_ref/1 -> udp_received_from_gumstix demux1/1
  [Psi_ref] -> Gyo Acc1/4
  Normal TrajGen/1(X_ref) -> Gyo Acc3/1
  Normal TrajGen/2(S_ref) -> Gyo Acc3/2
  Normal TrajGen/3(A_ref) -> Gyo Acc3/3
  Folding_scenario_ON/1 -> [Folding_scenario_ON]
  [Folding_scenario_ON] -> Switch/2
  Gyo Acc3/1 -> Switch/3
  [Folding_scenario_ON] -> Detect Fall Nonpositive/1
  Detect Fall Nonpositive/1 -> Normal TrajGen/3(Reset with X0)
  [V_ref] -> Gyo Acc1/2
  Constant/1 -> Gyo Acc1/3
  X0/1 -> Full TrajGen/2(X0), Scenario TrajGen/2(X0), Normal TrajGen/2(X0)
  udp_received_from_gumstix demux1/3 -> [V_ref]
  [X_ref] -> Scenario TrajGen/1(Ref)
  Scenario TrajGen/1(X_ref) -> Gyo Acc2/1, Gyo Acc1/1
  [Folding_scenario_ON] -> Detect Rise Positive/1
  Detect Rise Positive/1 -> Scenario TrajGen/3(Reset with X0)
  Scenario TrajGen/2(S_ref) -> Gyo Acc2/2
  Scenario TrajGen/3(A_ref) -> Gyo Acc2/3
  speed_ctrl_ON/1 -> [speed_ctrl_ON]
  [speed_ctrl_ON] -> Switch1/2
  [Psi_ref] -> Gyo Acc3/4
  Switch1/1 -> Switch/1
  Gyo Acc1/1 -> Switch1/1
  Gyo Acc2/1 -> Switch1/3
  [Psi_ref] -> Gyo Acc2/4
  Manual Switch/1 -> X_ref_FF/1
  Switch/1 -> Manual Switch/2
  Full TrajGen/1(X_ref) -> Gyo Acc4/1
  Full TrajGen/2(S_ref) -> Gyo Acc4/2
  Full TrajGen/3(A_ref) -> Gyo Acc4/3
  Gyo Acc4/1 -> Manual Switch/1
  [Psi_ref] -> Gyo Acc4/4
  [X_ref] -> Full TrajGen/1(Ref)
  [Folding_scenario_ON] -> Full TrajGen/3(Reset with X0)

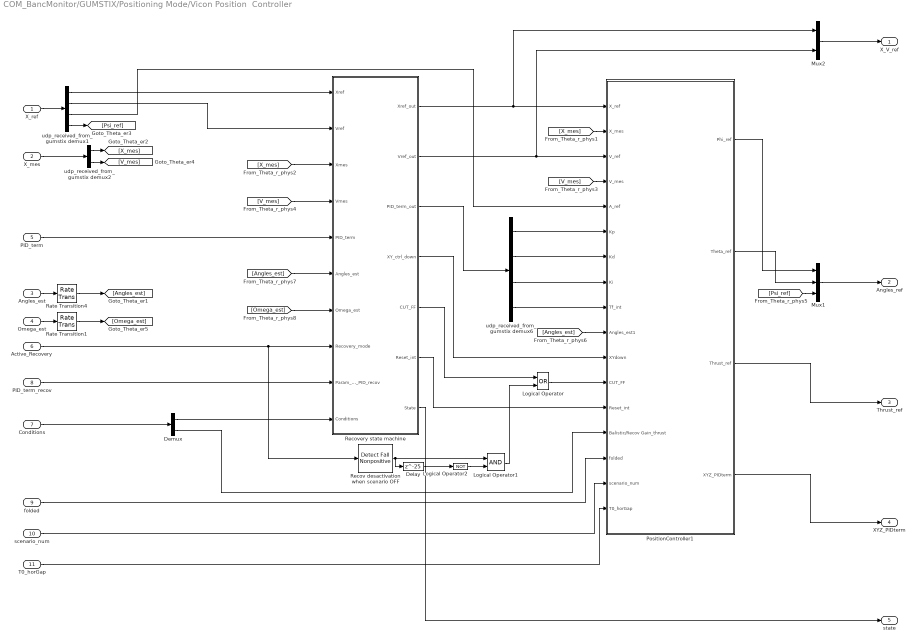
== system COM_BancMonitor/GUMSTIX/Positioning Mode/Vicon Position  Controller ==
  X_ref : Inport
  X_mes : Inport  Port=2
  Angles_est : Inport  Port=3
  Omega_est : Inport  Port=4
  PID_term : Inport  Port=5
  Active_Recovery : Inport  Port=6
  Conditions : Inport  Port=7
  PID_term_recov : Inport  Port=8
  folded : Inport  Port=9
  scenario_num : Inport  Port=10
  T0_horGap : Inport  Port=11
  Delay : Delay  DelayLength=25  InitialCondition=0
  Demux : Demux  Outputs=[4 2]
  Logical Operator : Logic  Operator=OR  AllPortsSameDT=off  OutDataTypeStr=boolean
  Logical Operator1 : Logic  AllPortsSameDT=off  OutDataTypeStr=boolean
  Logical Operator2 : Logic  Operator=NOT  AllPortsSameDT=off  OutDataTypeStr=boolean
  Mux1 : Mux  Inputs=[1 1 1]
  Mux2 : Mux  Inputs=2
  PositionController1 : Subsystem
  Rate Transition1 : RateTransition  OutPortSampleTime=Ts_PositionLoop
  Rate Transition4 : RateTransition  OutPortSampleTime=Ts_PositionLoop
  Recov desactivation when scenario OFF : simulink/Logic and Bit Operations/Detect Fall Nonpositive  vinit=1  InputProcessing=Inherited  OutDataTypeStr=boolean
  Recovery state machine : Subsystem
  udp_received_from_gumstix demux1 : Demux  Outputs=[3 3 3 1]
  udp_received_from_gumstix demux2 : Demux  Outputs=[3 3]
  udp_received_from_gumstix demux6 : Demux  Outputs=[3 3 3 3]
  X_V_ref : Outport  InitialOutput=eye(3, 3)
  Angles_ref : Outport  Port=2  InitialOutput=eye(3, 3)
  Thrust_ref : Outport  Port=3  InitialOutput=0
  XYZ_PIDterm : Outport  Port=4  InitialOutput=0
  state : Outport  Port=5  InitialOutput=0
  wires:
  Mux1/1 -> Angles_ref/1
  PositionController1/3(Thrust_ref) -> Thrust_ref/1
  X_ref/1 -> udp_received_from_gumstix demux1/1
  Angles_est/1 -> Rate Transition4/1
  udp_received_from_gumstix demux2/1 -> [X_mes]
  udp_received_from_gumstix demux2/2 -> [V_mes]
  udp_received_from_gumstix demux1/4 -> [Psi_ref]
  PositionController1/1(Phi_ref) -> Mux1/1
  PositionController1/2(Theta_ref) -> Mux1/2
  [Psi_ref] -> Mux1/3
  udp_received_from_gumstix demux6/1 -> PositionController1/6(Kp)
  udp_received_from_gumstix demux6/2 -> PositionController1/7(Kd)
  udp_received_from_gumstix demux6/3 -> PositionController1/8(Ki)
  udp_received_from_gumstix demux6/4 -> PositionController1/9(Tf_int)
  udp_received_from_gumstix demux1/3 -> PositionController1/5(A_ref)
  Recovery state machine/4(XY_ctrl_down) -> PositionController1/11(XYdown)
  udp_received_from_gumstix demux1/1 -> Recovery state machine/1(Xref)
  [X_mes] -> Recovery state machine/3(Xmes)
  [V_mes] -> Recovery state machine/4(Vmes)
  PID_term/1 -> Recovery state machine/5(PID_term)
  Active_Recovery/1 -> Recov desactivation when scenario OFF/1, Recovery state machine/8(Recovery_mode)
  Recovery state machine/3(PID_term_out) -> udp_received_from_gumstix demux6/1
  Recovery state machine/2(Vref_out) -> PositionController1/3(V_ref), Mux2/2
  Recovery state machine/1(Xref_out) -> Mux2/1, PositionController1/1(X_ref)
  udp_received_from_gumstix demux1/2 -> Recovery state machine/2(Vref)
  X_mes/1 -> udp_received_from_gumstix demux2/1
  [X_mes] -> PositionController1/2(X_mes)
  [V_mes] -> PositionController1/4(V_mes)
  Rate Transition4/1 -> [Angles_est]
  [Angles_est] -> PositionController1/10(Angles_est1)
  [Angles_est] -> Recovery state machine/6(Angles_est)
  Omega_est/1 -> Rate Transition1/1
  Rate Transition1/1 -> [Omega_est]
  [Omega_est] -> Recovery state machine/7(Omega_est)
  Recovery state machine/6(Reset_int) -> PositionController1/13(Reset_int)
  Mux2/1 -> X_V_ref/1
  PositionController1/4(XYZ_PIDterm) -> XYZ_PIDterm/1
  Recovery state machine/7(State) -> state/1
  Demux/1 -> Recovery state machine/10(Conditions)
  Conditions/1 -> Demux/1
  Demux/2 -> PositionController1/14(Balistic/Recov Gain_thrust)
  folded/1 -> PositionController1/15(folded)
  Logical Operator/1 -> PositionController1/12(CUT_FF)
  Recovery state machine/5(CUT_FF) -> Logical Operator/1
  Logical Operator1/1 -> Logical Operator/2
  Delay/1 -> Logical Operator2/1
  Recov desactivation when scenario OFF/1 -> Delay/1, Logical Operator1/1
  Logical Operator2/1 -> Logical Operator1/2
  scenario_num/1 -> PositionController1/16(scenario_num)
  T0_horGap/1 -> PositionController1/17(T0_horGap)
  PID_term_recov/1 -> Recovery state machine/9(Param_Pos_PID_recov)

== system COM_BancMonitor/GUMSTIX/Torques  Disturbances/Triggered Subsystem ==
  TorquesDist Mag : Inport
  Dt : Inport  Port=2
  Enable : EnablePort  StatesWhenEnabling=reset
  Constant : Constant  OutDataTypeStr=single
  Discrete-Time Integrator : DiscreteIntegrator  SampleTime=-1  ICPrevOutput=DiscIntNeverNeededParam  ICPrevScaledInput=DiscIntNeverNeededParam
  MATLAB Function : MATLAB Function  TreatAsAtomicUnit=on
  DisturbTorques : Outport  InitialOutput=[0 0 0]
  wires:
  TorquesDist Mag/1 -> MATLAB Function/1(TorquesDistMag)
  Constant/1 -> Discrete-Time Integrator/1
  Discrete-Time Integrator/1 -> MATLAB Function/2(Time)
  Dt/1 -> MATLAB Function/3(Dt)
  MATLAB Function/1(TorquesDist) -> DisturbTorques/1

== system COM_BancMonitor/GUMSTIX/Torques  Disturbances/Triggered Subsystem1 ==
  TorquesDist Mag : Inport
  Dt : Inport  Port=2
  Enable : EnablePort  StatesWhenEnabling=reset
  Constant : Constant  OutDataTypeStr=single
  Discrete-Time Integrator : DiscreteIntegrator  SampleTime=-1  ICPrevOutput=DiscIntNeverNeededParam  ICPrevScaledInput=DiscIntNeverNeededParam
  MATLAB Function : MATLAB Function  TreatAsAtomicUnit=on
  DisturbTorques : Outport  InitialOutput=[0 0 0]
  wires:
  TorquesDist Mag/1 -> MATLAB Function/1(TorquesDistMag)
  Constant/1 -> Discrete-Time Integrator/1
  Discrete-Time Integrator/1 -> MATLAB Function/2(Time)
  Dt/1 -> MATLAB Function/3(Dt)
  MATLAB Function/1(TorquesDist) -> DisturbTorques/1

== system COM_BancMonitor/GUMSTIX/Attitude controller/CTL_ATT_NL/Angles Disturbances ==
  Angles : Inport
  Dist_angles : Inport  Port=2
  Add : Sum
  Add1 : Sum
  Add2 : Sum
  Compare To Constant : simulink/Logic and Bit Operations/Compare To Constant  relop===  const=4  OutDataTypeStr=boolean
  Demux2 : Demux  Outputs=3
  Demux3 : Demux  Outputs=3
  Mux : Mux  Inputs=3
  Mux1 : Mux  Inputs=3
  Selector : Selector  InputPortWidth=5  IndexOptions=Index vector (dialog)  Indices=[1 2 3]  OutputSizes=1
  Selector2 : Selector  InputPortWidth=5  IndexOptions=Index vector (dialog)  Indices=4  OutputSizes=1
  Selector3 : Selector  InputPortWidth=5  IndexOptions=Index vector (dialog)  Indices=5  OutputSizes=1
  Triggered Subsystem : Subsystem  TreatAsAtomicUnit=on
  Angles_Out : Outport
  dist_angles_OUT : Outport  Port=2
  wires:
  Dist_angles/1 -> Selector2/1, Selector3/1, Selector/1
  Selector/1 -> Triggered Subsystem/1(AnglesDist Mag)
  Selector3/1 -> Mux1/3, Compare To Constant/1
  Demux2/1 -> Add/1
  Demux2/2 -> Add1/1
  Demux2/3 -> Add2/1
  Add/1 -> Mux/1
  Add1/1 -> Mux/2
  Add2/1 -> Mux/3
  Demux3/2 -> Add1/2
  Demux3/1 -> Add/2
  Demux3/3 -> Add2/2
  Selector2/1 -> Mux1/2, Triggered Subsystem/2(Dt)
  Angles/1 -> Demux2/1
  Mux/1 -> Angles_Out/1
  Compare To Constant/1 -> Triggered Subsystem/Enable
  Triggered Subsystem/1(DisturbAngles) -> Demux3/1, Mux1/1
  Mux1/1 -> dist_angles_OUT/1

== system COM_BancMonitor/GUMSTIX/Manual_Controller/RX Angles Ref  Generator/Rescale Pitch ==
  In : Inport
  Bias : Bias  Bias=-Bias_Scale
  Dead Zone : DeadZone  LowerValue=-DeadZone  UpperValue=DeadZone  SaturateOnIntegerOverflow=on
  Gain : Gain  Gain=Gscale
  Saturation : Saturate  UpperLimit=MaxOutput  LowerLimit=MinOutput
  Out : Outport
  wires:
  Bias/1 -> Dead Zone/1
  In/1 -> Bias/1
  Dead Zone/1 -> Gain/1
  Saturation/1 -> Out/1
  Gain/1 -> Saturation/1

== system COM_BancMonitor/GUMSTIX/Manual_Controller/RX Angles Ref  Generator/Rescale Roll ==
  In : Inport
  Bias : Bias  Bias=-Bias_Scale
  Dead Zone : DeadZone  LowerValue=-DeadZone  UpperValue=DeadZone  SaturateOnIntegerOverflow=on
  Gain : Gain  Gain=Gscale
  Saturation : Saturate  UpperLimit=MaxOutput  LowerLimit=MinOutput
  Out : Outport
  wires:
  Gain/1 -> Saturation/1
  Saturation/1 -> Out/1
  Dead Zone/1 -> Gain/1
  In/1 -> Bias/1
  Bias/1 -> Dead Zone/1

== system COM_BancMonitor/GUMSTIX/Manual_Controller/RX Angles Ref  Generator/Rescale Yaw ==
  In : Inport
  Bias : Bias  Bias=-Bias_Scale
  Dead Zone : DeadZone  LowerValue=-DeadZone  UpperValue=DeadZone  SaturateOnIntegerOverflow=on
  Gain : Gain  Gain=Gscale
  Saturation : Saturate  UpperLimit=MaxOutput  LowerLimit=MinOutput
  Out : Outport
  wires:
  Gain/1 -> Saturation/1
  Saturation/1 -> Out/1
  Dead Zone/1 -> Gain/1
  In/1 -> Bias/1
  Bias/1 -> Dead Zone/1

== system COM_BancMonitor/GUMSTIX/Manual_Controller/RX Angles Ref  Generator/Rescale2 Throttle ==
  In : Inport
  Bias : Bias  Bias=-MinInput
  Gain : Gain  Gain=Gscale
  Saturation : Saturate  UpperLimit=MaxOutput  LowerLimit=MinOutput
  Out : Outport
  wires:
  Bias/1 -> Gain/1
  In/1 -> Bias/1
  Saturation/1 -> Out/1
  Gain/1 -> Saturation/1

== system COM_BancMonitor/GUMSTIX/Positioning Mode/ClosedLoop Position SetPoint Generator/Full TrajGen ==
  Ref : Inport
  X0 : Inport  Port=2
  Reset with X0 : Inport  Port=3
  Add : Sum  Inputs=+-
  Gain : Gain  Gain=2*Tau.^2
  Gain1 : Gain  Gain=3*Tau
  Gain3 : Gain  Gain=1./Tau.^3
  Rate Transition3 : RateTransition  Deterministic=off
  Saturation : Saturate  UpperLimit=Xmax  LowerLimit=Xmin
  Selector1 : Selector  InputPortWidth=6  IndexOptions=Index vector (dialog)  Indices=[1 2 3]  OutputSizes=1
  Selector2 : Selector  InputPortWidth=6  IndexOptions=Index vector (dialog)  Indices=[4 5 6]  OutputSizes=1
  Sum : Sum  Inputs=+|+|+
  dA : DiscreteIntegrator  SampleTime=Ts_Filter  LimitOutput=on  UpperSaturationLimit=Amax  LowerSaturationLimit=Amin  ICPrevOutput=DiscIntNeverNeededParam  ICPrevScaledInput=DiscIntNeverNeededParam
  dV : DiscreteIntegrator  ExternalReset=rising  InitialConditionSource=external  SampleTime=Ts_Filter  LimitOutput=on  UpperSaturationLimit=Smax  LowerSaturationLimit=Smin  ICPrevOutput=DiscIntNeverNeededParam  ICPrevScaledInput=DiscIntNeverNeededParam
  dX : DiscreteIntegrator  ExternalReset=rising  InitialConditionSource=external  SampleTime=Ts_Filter  LimitOutput=on  UpperSaturationLimit=Xmax  LowerSaturationLimit=Xmin  ICPrevOutput=DiscIntNeverNeededParam  ICPrevScaledInput=DiscIntNeverNeededParam
  X_ref : Outport
  S_ref : Outport  Port=2
  A_ref : Outport  Port=3
  wires:
  Saturation/1 -> Add/1
  Gain3/1 -> dA/1
  Gain/1 -> Sum/1
  Gain1/1 -> Sum/2
  Add/1 -> Gain3/1
  dV/1 -> S_ref/1, Gain1/1, dX/1
  dA/1 -> A_ref/1, Gain/1, dV/1
  dX/1 -> Sum/3, X_ref/1
  Ref/1 -> Saturation/1
  Reset with X0/1 -> Rate Transition3/1
  Sum/1 -> Add/2
  X0/1 -> Selector1/1, Selector2/1
  Selector1/1 -> dX/3
  Selector2/1 -> dV/3
  Rate Transition3/1 -> dV/2, dX/2

== system COM_BancMonitor/GUMSTIX/Positioning Mode/ClosedLoop Position SetPoint Generator/Normal TrajGen ==
  Ref : Inport
  X0 : Inport  Port=2
  Reset with X0 : Inport  Port=3
  Add : Sum  Inputs=+-
  Gain : Gain  Gain=2*Tau.^2
  Gain1 : Gain  Gain=3*Tau
  Gain3 : Gain  Gain=1./Tau.^3
  Rate Transition3 : RateTransition  Deterministic=off
  Saturation : Saturate  UpperLimit=Xmax  LowerLimit=Xmin
  Selector1 : Selector  InputPortWidth=6  IndexOptions=Index vector (dialog)  Indices=[1 2 3]  OutputSizes=1
  Selector2 : Selector  InputPortWidth=6  IndexOptions=Index vector (dialog)  Indices=[4 5 6]  OutputSizes=1
  Sum : Sum  Inputs=+|+|+
  dA : DiscreteIntegrator  ExternalReset=rising  SampleTime=Ts_Filter  LimitOutput=on  UpperSaturationLimit=Amax  LowerSaturationLimit=Amin  ICPrevOutput=DiscIntNeverNeededParam  ICPrevScaledInput=DiscIntNeverNeededParam
  dV : DiscreteIntegrator  ExternalReset=rising  InitialConditionSource=external  SampleTime=Ts_Filter  LimitOutput=on  UpperSaturationLimit=Smax  LowerSaturationLimit=Smin  ICPrevOutput=DiscIntNeverNeededParam  ICPrevScaledInput=DiscIntNeverNeededParam
  dX : DiscreteIntegrator  ExternalReset=rising  InitialConditionSource=external  SampleTime=Ts_Filter  LimitOutput=on  UpperSaturationLimit=Xmax  LowerSaturationLimit=Xmin  ICPrevOutput=DiscIntNeverNeededParam  ICPrevScaledInput=DiscIntNeverNeededParam
  X_ref : Outport
  S_ref : Outport  Port=2
  A_ref : Outport  Port=3
  wires:
  Saturation/1 -> Add/1
  Gain3/1 -> dA/1
  Gain/1 -> Sum/1
  Gain1/1 -> Sum/2
  Add/1 -> Gain3/1
  dV/1 -> S_ref/1, Gain1/1, dX/1
  dA/1 -> A_ref/1, Gain/1, dV/1
  dX/1 -> Sum/3, X_ref/1
  Ref/1 -> Saturation/1
  Reset with X0/1 -> Rate Transition3/1
  Sum/1 -> Add/2
  X0/1 -> Selector1/1, Selector2/1
  Selector1/1 -> dX/3
  Selector2/1 -> dV/3
  Rate Transition3/1 -> dV/2, dX/2, dA/2

== system COM_BancMonitor/GUMSTIX/Positioning Mode/ClosedLoop Position SetPoint Generator/Scenario TrajGen ==
  Ref : Inport
  X0 : Inport  Port=2
  Reset with X0 : Inport  Port=3
  Add : Sum  Inputs=+-
  Gain : Gain  Gain=2*Tau.^2
  Gain1 : Gain  Gain=3*Tau
  Gain3 : Gain  Gain=1./Tau.^3
  Rate Transition3 : RateTransition  Deterministic=off
  Saturation : Saturate  UpperLimit=Xmax  LowerLimit=Xmin
  Selector1 : Selector  InputPortWidth=6  IndexOptions=Index vector (dialog)  Indices=[1 2 3]  OutputSizes=1
  Selector2 : Selector  InputPortWidth=6  IndexOptions=Index vector (dialog)  Indices=[4 5 6]  OutputSizes=1
  Sum : Sum  Inputs=+|+|+
  dA : DiscreteIntegrator  ExternalReset=rising  SampleTime=Ts_Filter  LimitOutput=on  UpperSaturationLimit=Amax  LowerSaturationLimit=Amin  ICPrevOutput=DiscIntNeverNeededParam  ICPrevScaledInput=DiscIntNeverNeededParam
  dV : DiscreteIntegrator  ExternalReset=rising  InitialConditionSource=external  SampleTime=Ts_Filter  LimitOutput=on  UpperSaturationLimit=Smax  LowerSaturationLimit=Smin  ICPrevOutput=DiscIntNeverNeededParam  ICPrevScaledInput=DiscIntNeverNeededParam
  dX : DiscreteIntegrator  ExternalReset=rising  InitialConditionSource=external  SampleTime=Ts_Filter  LimitOutput=on  UpperSaturationLimit=Xmax  LowerSaturationLimit=Xmin  ICPrevOutput=DiscIntNeverNeededParam  ICPrevScaledInput=DiscIntNeverNeededParam
  X_ref : Outport
  S_ref : Outport  Port=2
  A_ref : Outport  Port=3
  wires:
  Saturation/1 -> Add/1
  Gain3/1 -> dA/1
  Gain/1 -> Sum/1
  Gain1/1 -> Sum/2
  Add/1 -> Gain3/1
  dV/1 -> S_ref/1, Gain1/1, dX/1
  dA/1 -> A_ref/1, Gain/1, dV/1
  dX/1 -> Sum/3, X_ref/1
  Ref/1 -> Saturation/1
  Reset with X0/1 -> Rate Transition3/1
  Sum/1 -> Add/2
  X0/1 -> Selector1/1, Selector2/1
  Selector1/1 -> dX/3
  Selector2/1 -> dV/3
  Rate Transition3/1 -> dV/2, dX/2, dA/2
